simulink model "model_2021a"  (R2021a)
settings: Solver=VariableStepAuto  StartTime=0.0  StopTime=600  RelTol=1e-3
undefined symbols (not defined in the file or in its folder): National_Instruments, PCIe
libraries: sldrtlib x4
settings Model: Creator=lab  LastModifiedBy=zv210379d

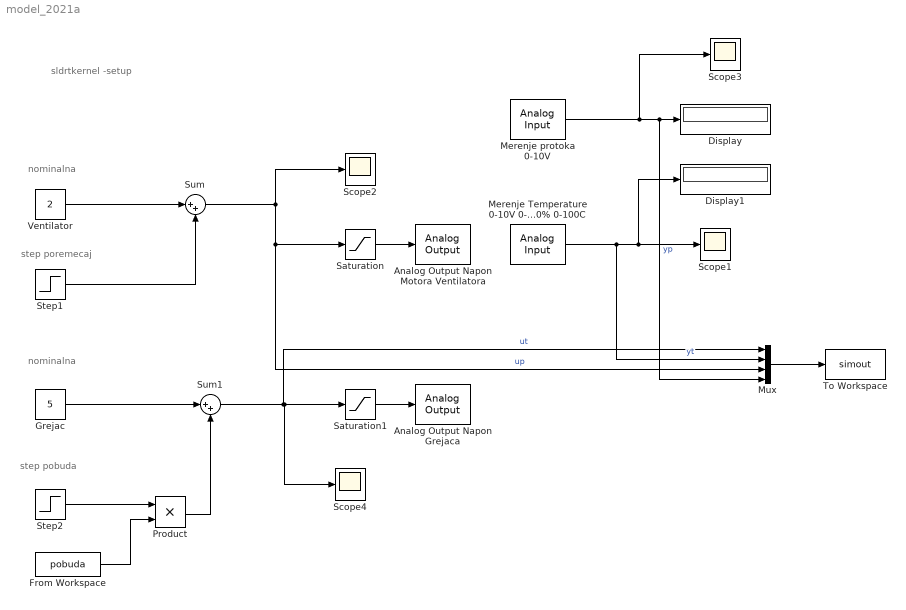
== system model_2021a ==
  note: step poremecaj
  note: step pobuda
  note: nominalna
  note: nominalna
  note: sldrtkernel -setup
  Analog Output Napon Grejaca : sldrtlib/Analog Output  SampleTime=0.01  MaxMissedTicks=10000  ShowMissedTicks=off  YieldWhenWaiting=off  DrvName=National_Instruments/PCIe-6323  DrvAddress=4294967295  DrvOptions=[0 0 0 0 0 0 0]  Channels=2  RangeMode=1  VoltRange=1  InitialValue=0  FinalValue=0
      settings: AttributesFormatString=National Instruments\nPCIe-6323 [auto]
  Analog Output Napon Motora Ventilatora : sldrtlib/Analog Output  SampleTime=0.01  MaxMissedTicks=10000  ShowMissedTicks=off  YieldWhenWaiting=off  DrvName=National_Instruments/PCIe-6323  DrvAddress=4294967295  DrvOptions=[0 0 0 0 0 0 0]  Channels=1  RangeMode=1  VoltRange=1  InitialValue=[]  FinalValue=[]
      settings: AttributesFormatString=National Instruments\nPCIe-6323 [auto]
  Display : Display
  Display1 : Display
  From Workspace : FromWorkspace  VariableName=pobuda
  Grejac : Constant  Value=5
  Merenje Temperature 0-10V 0-100% 0-100C : sldrtlib/Analog Input  SampleTime=0.01  MaxMissedTicks=10000  ShowMissedTicks=off  YieldWhenWaiting=off  DrvName=National_Instruments/PCIe-6323  DrvAddress=4294967295  DrvOptions=[0 0 0 0 0 0 0]  Channels=3  RangeMode=1  VoltRange=1  DataType=1
      settings: AttributesFormatString=National Instruments\nPCIe-6323 [auto]
  Merenje protoka 0-10V : sldrtlib/Analog Input  SampleTime=0.01  MaxMissedTicks=10000  ShowMissedTicks=off  YieldWhenWaiting=on  DrvName=National_Instruments/PCIe-6323  DrvAddress=4294967295  DrvOptions=[0 0 0 0 0 0 0]  Channels=6  RangeMode=1  VoltRange=1  DataType=1
      settings: AttributesFormatString=National Instruments\nPCIe-6323 [auto]
  Mux : Mux
  Product : Product
  Saturation : Saturate  UpperLimit=10  LowerLimit=0
  Saturation1 : Saturate  UpperLimit=10  LowerLimit=0
  Scope{1..4} (4 alike) : Scope
  Step1 : Step  Time=400  After=3  SampleTime=0
  Step2 : Step  Time=200  SampleTime=0
  Sum : Sum  Inputs=|++
  Sum1 : Sum  Inputs=|++
  To Workspace : ToWorkspace  VariableName=simout  SampleTime=0.01
  Ventilator : Constant  Value=2
  wires:
  Mux/1 -> To Workspace/1
  Saturation1/1 -> Analog Output Napon Grejaca/1
  Merenje protoka 0-10V/1 -> Display/1, Mux/4, Scope3/1  "yp"
  Saturation/1 -> Analog Output Napon Motora Ventilatora/1
  Merenje Temperature 0-10V 0-100% 0-100C/1 -> Mux/2, Display1/1, Scope1/1  "yt"
  Sum/1 -> Scope2/1, Mux/3, Saturation/1  "up"
  Grejac/1 -> Sum1/1
  Sum1/1 -> Mux/1, Scope4/1, Saturation1/1  "ut"
  Ventilator/1 -> Sum/1
  Step1/1 -> Sum/2
  Step2/1 -> Product/1
  Product/1 -> Sum1/2
  From Workspace/1 -> Product/2
